simulink model "R2G_ss_NE5kW_R2019a"  (R2019a)
settings: Solver=ode4  StartTime=0  StopTime=1200  FixedStep=simu.dt  MaxStep=0.1  RelTol=1e-3  EnableMultiTasking=on
undefined symbols (not defined in the file or in its folder): ess, gsc, mot, Pgen, Pgrid, Qgrid_lim, simu, Vdc, wsc
libraries: simulink x1
settings Model: Creator=mlawson  LastModifiedBy=eabrowning
settings SolverCC: ZeroCrossControl=DisableAll  AlgebraicLoopSolver=LineSearch  AutoInsertRateTranBlk=on
settings DataIOCC: SaveFormat=Array  SaveOutput=off  SaveTime=off  ReturnWorkspaceOutputs=off
settings OptimizationCC: LifeSpan=inf  SimCompilerOptimization=on
settings DebuggingCC: UnderspecifiedInitializationDetection=Classic  MergeDetectMultiDrivingBlocksExec=none  SolverPrmCheckMsg=warning  AllowSymbolicDim=off  StateNameClashWarn=warning  SFUnexpectedBacktrackingDiag=warning  SFNoUnconditionalDefaultTransitionDiag=warning  ArithmeticOperatorsInVariantConditions=warning
settings HardwareCC: ProdBitPerPointer=32  ProdBitPerSizeT=32  ProdBitPerPtrDiffT=32  ProdLargestAtomicFloat=None  ProdIntDivRoundTo=Undefined  ProdEndianess=Unspecified  ProdWordSize=32  ProdHWDeviceType=32-bit Generic
settings ModelReferenceCC: PropagateSignalLabelsOutOfModel=off
settings SFSimCC: SimUseLocalCustomCode=off
settings RTWCC: RTWUseLocalCustomCode=off
settings CodeAppCC: StateflowObjectComments=on
settings GRTTargetCC: TargetLangStandard=C89/C90 (ANSI)
settings ConfigComp: CovMetricSettings=dw  CovSaveCumulativeToWorkspaceVar=on  CovSaveSingleToWorkspaceVar=on  CovExternalEMLEnable=off  CovSFcnEnable=off
settings SimscapeCC: SimscapeNormalizeSystem=off
settings ConfigurationSet: Description=SimMechanics 2G
settings ExplorerConfigSet: SimMechanicsOpenEditorOnUpdate=off  InternalSimMechanicsExplorerSettings="<ExplorerConfiguration><canonicalview>default</canonicalview><TilePanel><TileInfo><Tiles Columns=\"1\" Count=\"1\" Rows=\"1\"><Column Left=\"2\" Weight=\"1\"/><Column Left=\"1335\"/><Row Top=\"2\" Weight=\"1\"/><Row Top=\"911\"/><Tile Height=\"1\" Width=\"1\" X=\"0\" Y=\"0\"/></Tiles></TileInfo><SceneInfo><SceneViewer><BGColor><R>0.60000002384185791</R><G>0.60000002384185791</G><B>0.60000002384185791</B></BGColor><Camera><Position><X>365.37645888990272</X><Y>-369.82486814446582</Y><Z>359.64809521743916</Z></Position><Center><X>-6.7351450971904585</X><Y>2.2867358426280204</Y><Z>-12.463508769654169</Z></Center><Up><X>-0.40824829046386307</X><Y>0.40824829046386307</Y><Z>0.81649658092772615</Z></Up><Left>-57.820127362122818</Left><Right>57.820127362122818</Right><Bottom>-38.308817187253304</Bottom><Top>38.308817187253304</Top></Camera></SceneViewer></SceneInfo></TilePanel></ExplorerConfiguration>"

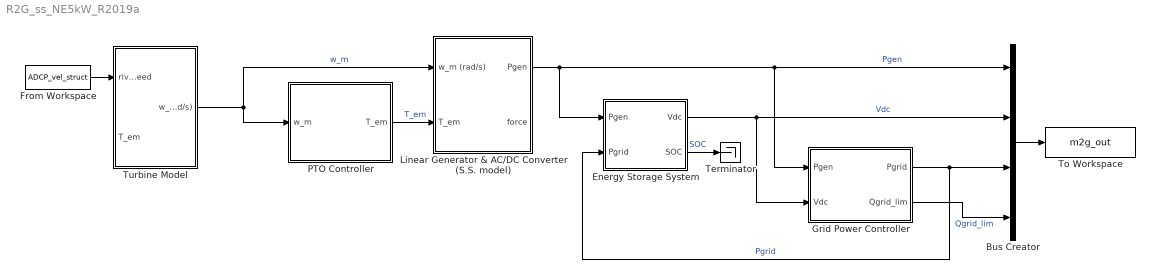
== system R2G_ss_NE5kW_R2019a ==
  Bus Creator : BusCreator  Inputs=Pgen,Vdc,Pgrid,Qgrid_lim
  Energy Storage System : Subsystem  mask{SOC_0=ess.SOC_0, Csoc=ess.Csoc, SOC_LUT=ess.SOC_LUT, Voc_LUT=ess.Voc_LUT, eff=ess.eff}
      mask prompts: SOC_0 "Initial SOC"; Csoc "SOC equivalent capacitance (C):"; SOC_LUT "SOC LUT"; Voc_LUT "Voc LUT"; eff "Efficiency"
      mask DialogControl DescTextVar_copy Prompt: Uses a generalized energy storage model.
      mask DialogControl ParamGroupVar Prompt: Energy Storage Parameters
  From Workspace : FromWorkspace  VariableName=ADCP_vel_struct  OutDataTypeStr=double  OutputAfterFinalValue=Holding final value
  Grid Power Controller : Subsystem  mask{Tavg=gsc.Tavg, Vmag=gsc.Vmag, Ilim=gsc.Ilim, Prated=gsc.Prated, Vdc_nom=ess.Vdc_0, Vdc_del=ess.Vdc_del, kp_v=gsc.kp, ki_v=gsc.ki}
      mask prompts: Tavg "Averaging Time Constant (s):"; Vmag "Grid voltage magnitude (V):"; Ilim "GSC current limit (A):"; Prated "GSC rated power (W):"; Vdc_nom "DC link nominal voltage (V):"; Vdc_del "DC link voltage deviation maximum (V):"; kp_v "Voltage regulator proportional gain:"; ki_v "Voltage regulator integral gain:"
  Linear Generator & AC/DC Converter (S.S. model) : Subsystem  mask{ptoSim=mot}
      mask prompts: ptoSim "Machine Name"
  PTO Controller : Subsystem
  Terminator : Terminator
  To Workspace : ToWorkspace  VariableName=m2g_out  SaveFormat=Timeseries  SampleTime=-1
  Turbine Model : Subsystem
  wires:
  Linear Generator & AC/DC Converter (S.S. model)/1(Pgen) -> Bus Creator/1, Grid Power Controller/1(Pgen), Energy Storage System/1(Pgen)  "Pgen"
  Grid Power Controller/1(Pgrid) -> Bus Creator/3, Energy Storage System/2(Pgrid)  "Pgrid"
  Grid Power Controller/2(Qgrid_lim) -> Bus Creator/4  "Qgrid_lim"
  Energy Storage System/1(Vdc) -> Grid Power Controller/2(Vdc), Bus Creator/2  "Vdc"
  PTO Controller/1(T_em) -> Linear Generator & AC/DC Converter (S.S. model)/2(T_em)  "T_em"
  Bus Creator/1 -> To Workspace/1
  Energy Storage System/2(SOC) -> Terminator/1  "SOC"
  Turbine Model/1(w_m (rad/s)) -> Linear Generator & AC/DC Converter (S.S. model)/1(w_m (rad/s)), PTO Controller/1(w_m)  "w_m"
  From Workspace/1 -> Turbine Model/1(river speed)

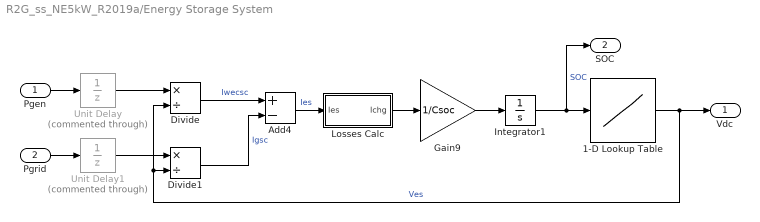
== system R2G_ss_NE5kW_R2019a/Energy Storage System ==
  Pgen : Inport
  Pgrid : Inport  Port=2
  1-D Lookup Table : Lookup_n-D  NumberOfTableDimensions=1  BreakpointsForDimension1=SOC_LUT  Table=Voc_LUT  InternalRulePriority=Speed  RndMeth=Simplest  InputSameDT=on
  Add4 : Sum  Inputs=+-
  Divide : Product  Inputs=*/
  Divide1 : Product  Inputs=*/
  Gain9 : Gain  Gain=1/Csoc
  Integrator1 : Integrator  InitialCondition=SOC_0
  Losses Calc : Subsystem
  Unit Delay : UnitDelay  Commented=through  SampleTime=-1  HasFrameUpgradeWarning=on
  Unit Delay1 : UnitDelay  Commented=through  SampleTime=-1  HasFrameUpgradeWarning=on
  Vdc : Outport  VectorParamsAs1DForOutWhenUnconnected=on
  SOC : Outport  Port=2  VectorParamsAs1DForOutWhenUnconnected=on
  wires:
  Unit Delay1/1 -> Divide1/1
  Unit Delay/1 -> Divide/1
  Pgrid/1 -> Unit Delay1/1
  Divide1/1 -> Add4/2  "Igsc"
  Gain9/1 -> Integrator1/1
  Divide/1 -> Add4/1  "Iwecsc"
  Pgen/1 -> Unit Delay/1
  Integrator1/1 -> SOC/1, 1-D Lookup Table/1  "SOC"
  1-D Lookup Table/1 -> Divide/2, Divide1/2, Vdc/1  "Ves"
  Add4/1 -> Losses Calc/1(Ies)  "Ies"
  Losses Calc/1(Ichg) -> Gain9/1

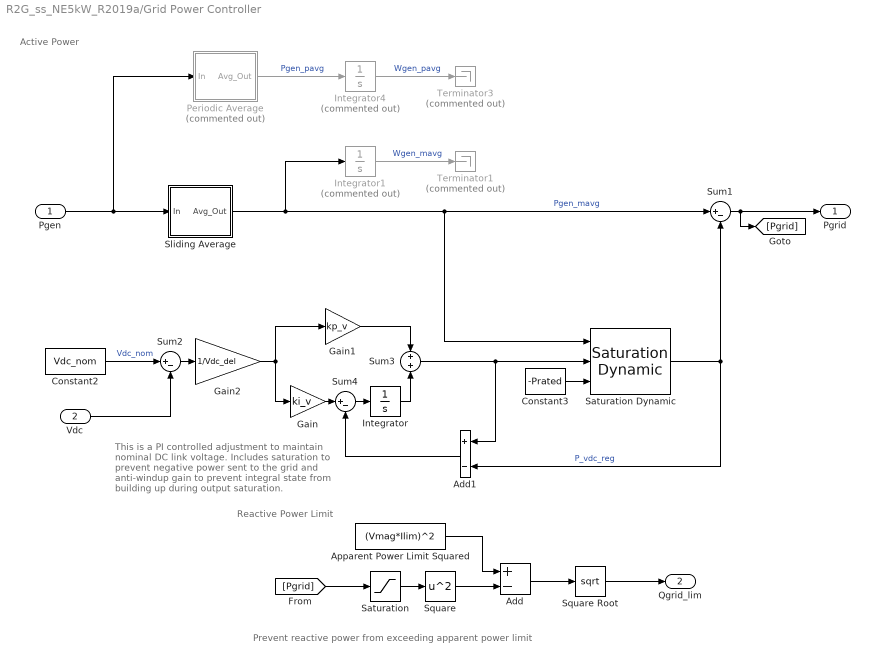
== system R2G_ss_NE5kW_R2019a/Grid Power Controller ==
  note: This is a PI controlled adjustment to maintain nominal DC link voltage. Includes saturation to prevent negative power sent to the grid and anti-windup gain to prevent integral state from building up during output saturation.
  note: Reactive Power Limit
  note: Active Power
  note: Prevent reactive power from exceeding apparent power limit
  Pgen : Inport
  Vdc : Inport  Port=2
  Add : Sum  Inputs=+-
  Add1 : Sum  Inputs=+-
  Apparent Power Limit Squared : Constant  Value=(Vmag*Ilim)^2
  Constant2 : Constant  Value=Vdc_nom
  Constant3 : Constant  Value=-Prated
  Gain : Gain  Gain=ki_v
  Gain1 : Gain  Gain=kp_v
  Gain2 : Gain  Gain=1/Vdc_del
  Integrator : Integrator
  Integrator1 : Integrator  Commented=on
  Integrator4 : Integrator  Commented=on
  Periodic Average : Subsystem  Commented=on  mask{Tsample=Tavg}
      mask prompts: Tsample "Sampling Period (s):"
  Saturation : Saturate  UpperLimit=Vmag*Ilim  LowerLimit=-Vmag*Ilim
  Saturation Dynamic : simulink/Discontinuities/Saturation Dynamic  OutMin=[]  OutMax=[]  OutDataTypeStr=Inherit: Same as second input  OutDataType=fixdt(1, 16)  OutScaling=2^-10  DoSatur=off
  Sliding Average : Subsystem  mask{Tsample=Tavg, dt=simu.dt}
      mask prompts: Tsample "Sampling Period (s):"; dt "Simulation Time Step (s):"
  Square : Math  Operator=square  SaturateOnIntegerOverflow=on
  Square Root : Sqrt  SaturateOnIntegerOverflow=on
  Sum1 : Sum  Inputs=|+-
  Sum2 : Sum  Inputs=|+-
  Sum3 : Sum
  Sum4 : Sum  Inputs=|+-
  Terminator1 : Terminator  Commented=on
  Terminator3 : Terminator  Commented=on
  Pgrid : Outport  VectorParamsAs1DForOutWhenUnconnected=on
  Qgrid_lim : Outport  Port=2  VectorParamsAs1DForOutWhenUnconnected=on
  wires:
  Pgen/1 -> Periodic Average/1(In), Sliding Average/1(In)
  Integrator4/1 -> Terminator3/1  "Wgen_pavg"
  Integrator1/1 -> Terminator1/1  "Wgen_mavg"
  Sliding Average/1(Avg_Out) -> Saturation Dynamic/1, Sum1/1, Integrator1/1  "Pgen_mavg"
  Periodic Average/1(Avg_Out) -> Integrator4/1  "Pgen_pavg"
  Add/1 -> Square Root/1
  Square/1 -> Add/2
  Saturation/1 -> Square/1
  Square Root/1 -> Qgrid_lim/1
  Apparent Power Limit Squared/1 -> Add/1
  Sum1/1 -> [Pgrid], Pgrid/1
  [Pgrid] -> Saturation/1
  Constant2/1 -> Sum2/1  "Vdc_nom"
  Constant3/1 -> Saturation Dynamic/3
  Sum3/1 -> Add1/1, Saturation Dynamic/2
  Gain1/1 -> Sum3/1
  Integrator/1 -> Sum3/2
  Saturation Dynamic/1 -> Add1/2, Sum1/2  "P_vdc_reg"
  Vdc/1 -> Sum2/2
  Sum2/1 -> Gain2/1
  Gain2/1 -> Gain1/1, Gain/1
  Gain/1 -> Sum4/1
  Sum4/1 -> Integrator/1
  Add1/1 -> Sum4/2

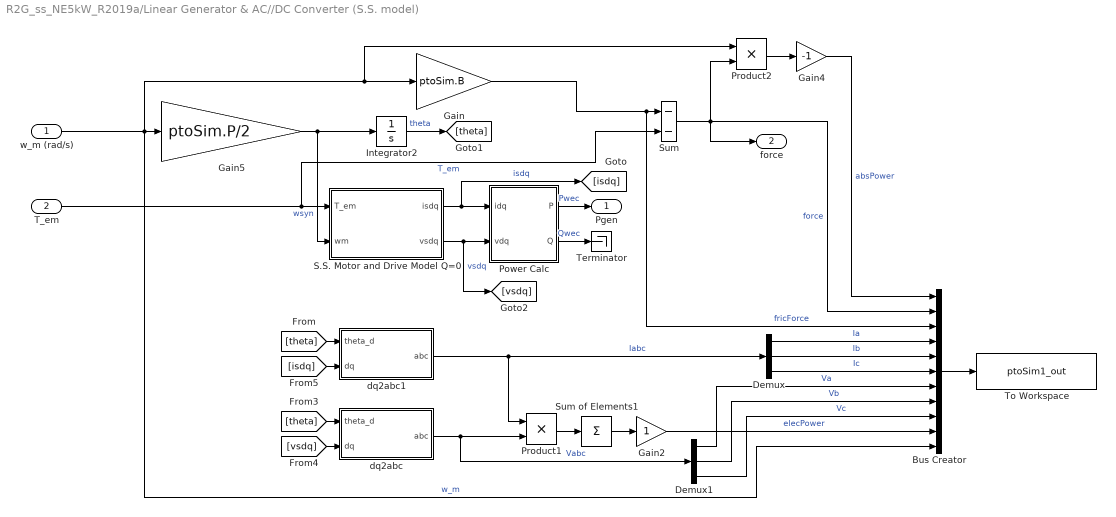
== system R2G_ss_NE5kW_R2019a/Linear Generator & AC//DC Converter (S.S. model) ==
  w_m (rad/s) : Inport
  T_em : Inport  Port=2
  Bus Creator : BusCreator  Inputs=11
  Demux : Demux  Outputs=3
  Demux1 : Demux  Outputs=3
  Gain : Gain  Gain=ptoSim.B
  Gain2 : Gain
  Gain4 : Gain  Gain=-1
  Gain5 : Gain  Gain=ptoSim.P/2
  Integrator2 : Integrator  InitialCondition=ptoSim.theta_d_0
  Power Calc : Subsystem
  Product1 : Product
  Product2 : Product
  S.S. Motor and Drive Model Q=0 : Subsystem
  Sum : Sum  Inputs=--
  Sum of Elements1 : Sum  Inputs=+
  Terminator : Terminator
  To Workspace : ToWorkspace  VariableName=ptoSim1_out  SaveFormat=Structure With Time  SampleTime=simu.dt
  dq2abc : Subsystem
  dq2abc1 : Subsystem
  Pgen : Outport  VectorParamsAs1DForOutWhenUnconnected=on
  force : Outport  Port=2  VectorParamsAs1DForOutWhenUnconnected=on
  wires:
  Gain/1 -> Sum/1, Bus Creator/3  "fricForce"
  S.S. Motor and Drive Model Q=0/2(vsdq) -> [vsdq], Power Calc/2(vdq)  "vsdq"
  Sum/1 -> Product2/2, force/1, Bus Creator/2  "force"
  Sum of Elements1/1 -> Gain2/1
  Integrator2/1 -> [theta]  "theta"
  w_m (rad/s)/1 -> Gain/1, Product2/1, Bus Creator/11, Gain5/1  "w_m"
  Gain2/1 -> Bus Creator/10  "elecPower"
  Product1/1 -> Sum of Elements1/1
  dq2abc/1(abc) -> Demux1/1, Product1/2  "Vabc"
  Demux1/3 -> Bus Creator/9  "Vc"
  Demux1/2 -> Bus Creator/8  "Vb"
  Demux/3 -> Bus Creator/6  "Ic"
  Gain5/1 -> Integrator2/1, S.S. Motor and Drive Model Q=0/2(wm)  "wsyn"
  Demux1/1 -> Bus Creator/7  "Va"
  Demux/1 -> Bus Creator/4  "Ia"
  S.S. Motor and Drive Model Q=0/1(isdq) -> Power Calc/1(idq), [isdq]  "isdq"
  Bus Creator/1 -> To Workspace/1
  Demux/2 -> Bus Creator/5  "Ib"
  dq2abc1/1(abc) -> Product1/1, Demux/1  "Iabc"
  Gain4/1 -> Bus Creator/1  "absPower"
  Product2/1 -> Gain4/1
  Power Calc/2(Q) -> Terminator/1  "Qwec"
  Power Calc/1(P) -> Pgen/1  "Pwec"
  [theta] -> dq2abc1/1(theta_d)
  [theta] -> dq2abc/1(theta_d)
  [vsdq] -> dq2abc/2(dq)
  [isdq] -> dq2abc1/2(dq)
  T_em/1 -> S.S. Motor and Drive Model Q=0/1(T_em), Sum/2  "T_em"

== system R2G_ss_NE5kW_R2019a/PTO Controller ==
  w_m : Inport
  Current-based force limit : Saturate  UpperLimit=wsc.Fpto_lim  LowerLimit=-wsc.Fpto_lim
  Gain1 : Gain  Gain=wsc.Bdamp
  T_em : Outport  VectorParamsAs1DForOutWhenUnconnected=on
  wires:
  Gain1/1 -> Current-based force limit/1  "T_em"
  w_m/1 -> Gain1/1
  Current-based force limit/1 -> T_em/1

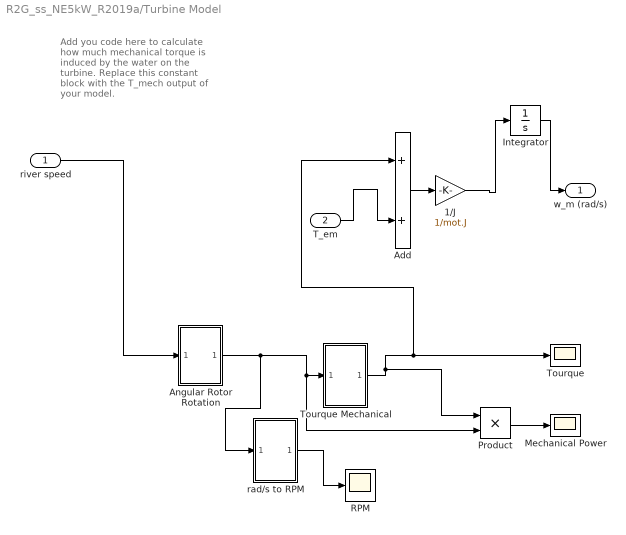
== system R2G_ss_NE5kW_R2019a/Turbine Model ==
  note: Add you code here to calculate how much mechanical torque is induced by the water on the turbine. Replace this constant block with the T_mech output of your model.
  river speed : Inport
  T_em : Inport  Port=2
  " Tourque Mechanical" : Subsystem
  1/J : Gain  Gain=1/mot.J
  Add : Sum
  Angular Rotor Rotation : Subsystem
  Integrator : Integrator
  Mechanical Power : Scope
  Product : Product
  RPM : Scope
  Tourque : Scope
  rad/s to RPM : Subsystem
  w_m (rad/s) : Outport  VectorParamsAs1DForOutWhenUnconnected=on
  wires:
  1/J/1 -> Integrator/1
  Add/1 -> 1/J/1
  rad/s to RPM/1(Out1) -> RPM/1
  Angular Rotor Rotation/1(Out1) -> rad/s to RPM/1(In1), Product/2, " Tourque Mechanical"/1(In1)
  river speed/1 -> Angular Rotor Rotation/1(In1)
  Product/1 -> Mechanical Power/1
  " Tourque Mechanical"/1(Out1) -> Add/1, Tourque/1, Product/1
  T_em/1 -> Add/2
  Integrator/1 -> w_m (rad/s)/1

== system R2G_ss_NE5kW_R2019a/Energy Storage System/Losses Calc ==
  Ies : Inport
  Gain1 : Gain  Gain=1/eff
  Gain2 : Gain  Gain=eff
  Switch : Switch  Criteria=u2 > Threshold
  Ichg : Outport  VectorParamsAs1DForOutWhenUnconnected=on
  wires:
  Ies/1 -> Gain1/1, Gain2/1, Switch/2
  Switch/1 -> Ichg/1
  Gain2/1 -> Switch/1
  Gain1/1 -> Switch/3

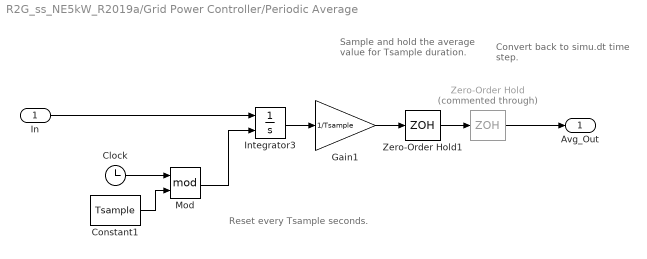
== system R2G_ss_NE5kW_R2019a/Grid Power Controller/Periodic Average ==
  note: Reset every Tsample seconds.
  note: Convert back to simu.dt time step.
  note: Sample and hold the average value for Tsample duration.
  In : Inport
  Clock : Clock
  Constant1 : Constant  Value=Tsample
  Gain1 : Gain  Gain=1/Tsample
  Integrator3 : Integrator  ExternalReset=rising
  Mod : Math  Operator=mod  OutputSignalType=real  SaturateOnIntegerOverflow=on
  Zero-Order Hold : ZeroOrderHold  Commented=through  SampleTime=simu.dt
  Zero-Order Hold1 : ZeroOrderHold  SampleTime=Tsample
  Avg_Out : Outport  VectorParamsAs1DForOutWhenUnconnected=on
  wires:
  Zero-Order Hold/1 -> Avg_Out/1
  Mod/1 -> Integrator3/2
  Zero-Order Hold1/1 -> Zero-Order Hold/1
  Clock/1 -> Mod/1
  Gain1/1 -> Zero-Order Hold1/1
  Integrator3/1 -> Gain1/1
  In/1 -> Integrator3/1
  Constant1/1 -> Mod/2

== system R2G_ss_NE5kW_R2019a/Grid Power Controller/Sliding Average ==
  In : Inport
  Discrete FIR Filter : DiscreteFir  Coefficients=ones(1,round(Tsample/dt))/round(Tsample/dt)  SampleTime=dt
  Avg_Out : Outport  VectorParamsAs1DForOutWhenUnconnected=on
  wires:
  In/1 -> Discrete FIR Filter/1
  Discrete FIR Filter/1 -> Avg_Out/1

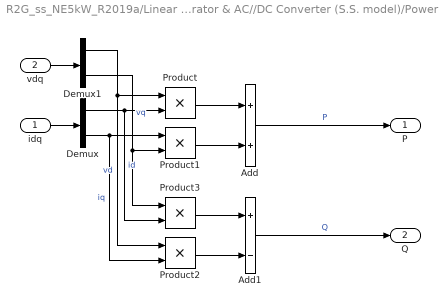
== system R2G_ss_NE5kW_R2019a/Linear Generator & AC//DC Converter (S.S. model)/Power Calc ==
  idq : Inport
  vdq : Inport  Port=2
  Add : Sum
  Add1 : Sum  Inputs=+-
  Demux : Demux  Outputs=2
  Demux1 : Demux  Outputs=2
  Product{,1..3} (4 alike) : Product
  P : Outport  VectorParamsAs1DForOutWhenUnconnected=on
  Q : Outport  Port=2  VectorParamsAs1DForOutWhenUnconnected=on
  wires:
  Demux/1 -> Product3/2, Product/2  "id"
  Product1/1 -> Add/2
  Add1/1 -> Q/1  "Q"
  Demux1/2 -> Product1/2, Product3/1  "vq"
  Demux1/1 -> Product/1, Product2/1  "vd"
  Demux/2 -> Product2/2, Product1/1  "iq"
  Product3/1 -> Add1/1
  Product2/1 -> Add1/2
  Product/1 -> Add/1
  Add/1 -> P/1  "P"
  idq/1 -> Demux/1
  vdq/1 -> Demux1/1

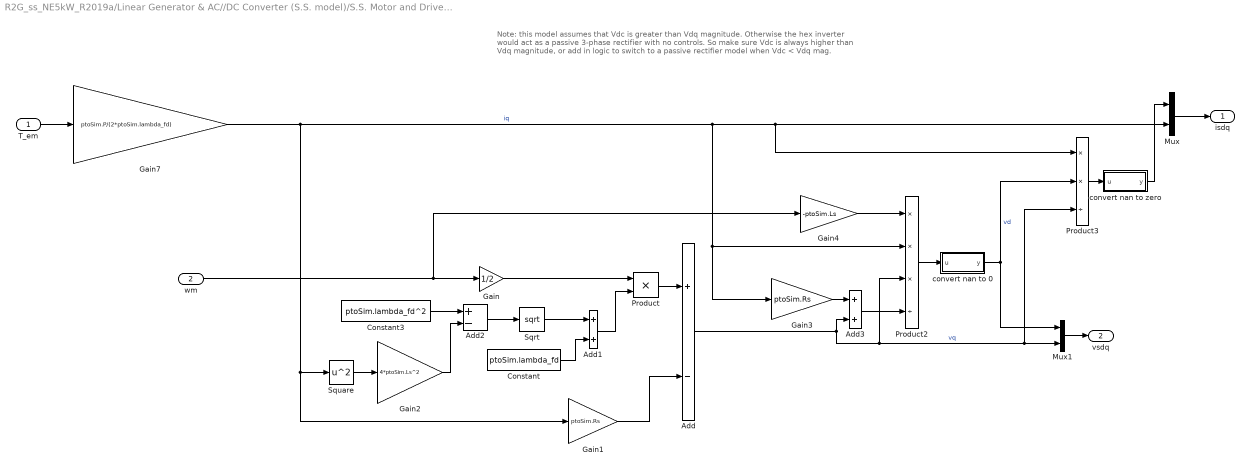
== system R2G_ss_NE5kW_R2019a/Linear Generator & AC//DC Converter (S.S. model)/S.S. Motor and Drive Model Q=0 ==
  note: Note: this model assumes that Vdc is greater than Vdq magnitude. Otherwise the hex inverter would act as a passive 3-phase rectifier with no controls. So make sure Vdc is always higher than Vdq magnitude, or add in logic to switch to a passive rectifier model when Vdc < Vdq mag.
  T_em : Inport
  wm : Inport  Port=2
  Add : Sum  Inputs=+-
  Add1 : Sum
  Add2 : Sum  Inputs=+-
  Add3 : Sum
  Constant : Constant  Value=ptoSim.lambda_fd
  Constant3 : Constant  Value=ptoSim.lambda_fd^2
  Gain : Gain  Gain=1/2
  Gain1 : Gain  Gain=ptoSim.Rs
  Gain2 : Gain  Gain=4*ptoSim.Ls^2
  Gain3 : Gain  Gain=ptoSim.Rs
  Gain4 : Gain  Gain=-ptoSim.Ls
  Gain7 : Gain  Gain=ptoSim.P/(2*ptoSim.lambda_fd)
  Mux : Mux  Inputs=2
  Mux1 : Mux  Inputs=2
  Product : Product
  Product2 : Product  Inputs=***/
  Product3 : Product  Inputs=**/
  Sqrt : Sqrt  SaturateOnIntegerOverflow=on
  Square : Math  Operator=square  SaturateOnIntegerOverflow=on
  convert nan to 0 : MATLAB Function  TreatAsAtomicUnit=on
  convert nan to zero : MATLAB Function  TreatAsAtomicUnit=on
  isdq : Outport  VectorParamsAs1DForOutWhenUnconnected=on
  vsdq : Outport  Port=2  VectorParamsAs1DForOutWhenUnconnected=on
  wires:
  T_em/1 -> Gain7/1
  Mux/1 -> isdq/1
  Mux1/1 -> vsdq/1
  Gain7/1 -> Product2/2, Gain3/1, Product3/1, Mux/2, Gain1/1, Square/1  "iq"
  Constant/1 -> Add1/2
  convert nan to 0/1(y) -> Product3/2, Mux1/1  "vd"
  Add/1 -> Product2/3, Product3/3, Mux1/2, Add3/2  "vq"
  convert nan to zero/1(y) -> Mux/1
  Gain1/1 -> Add/2
  Product/1 -> Add/1
  Gain/1 -> Product/1
  Add1/1 -> Product/2
  Sqrt/1 -> Add1/1
  Add2/1 -> Sqrt/1
  Constant3/1 -> Add2/1
  Gain2/1 -> Add2/2
  Product2/1 -> convert nan to 0/1(u)
  Add3/1 -> Product2/4
  Gain3/1 -> Add3/1
  Gain4/1 -> Product2/1
  Product3/1 -> convert nan to zero/1(u)
  Square/1 -> Gain2/1
  wm/1 -> Gain4/1, Gain/1

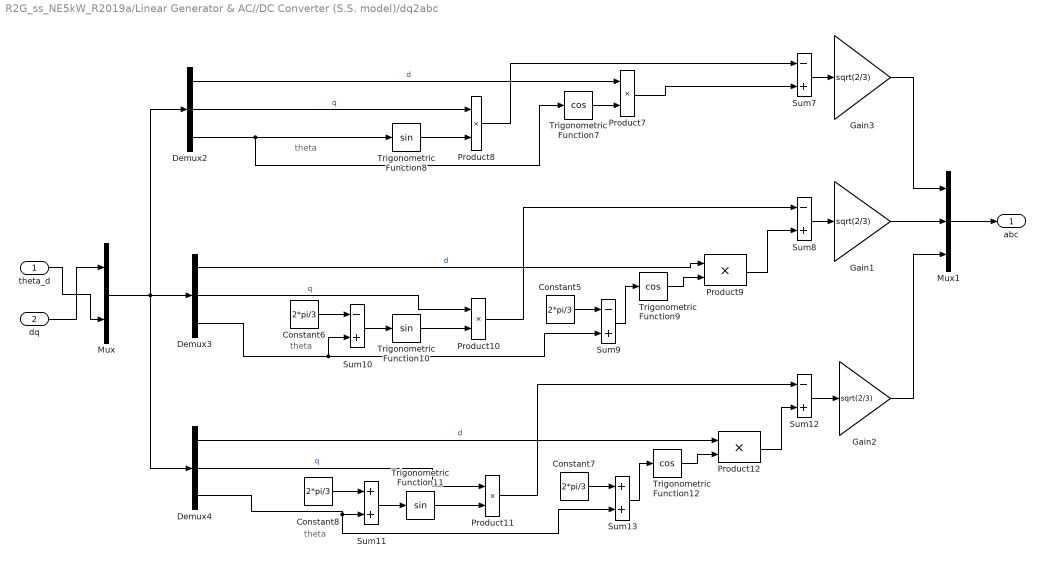
== system R2G_ss_NE5kW_R2019a/Linear Generator & AC//DC Converter (S.S. model)/dq2abc ==
  note: theta
  note: theta
  note: theta
  theta_d : Inport
  dq : Inport  Port=2
  Constant{5..8} (4 alike) : Constant  Value=2*pi/3
  Demux2 : Demux  Outputs=3
  Demux3 : Demux  Outputs=3
  Demux4 : Demux  Outputs=3
  Gain1 : Gain  Gain=sqrt(2/3)  SaturateOnIntegerOverflow=on  OutDataTypeStr=Inherit: Same as input  ParamDataTypeStr=Inherit: Same as input
  Gain2 : Gain  Gain=sqrt(2/3)  SaturateOnIntegerOverflow=on  OutDataTypeStr=Inherit: Same as input  ParamDataTypeStr=Inherit: Same as input
  Gain3 : Gain  Gain=sqrt(2/3)  SaturateOnIntegerOverflow=on  OutDataTypeStr=Inherit: Same as input  ParamDataTypeStr=Inherit: Same as input
  Mux : Mux  Inputs=2
  Mux1 : Mux  Inputs=3
  Product{7..12} (6 alike) : Product  SaturateOnIntegerOverflow=on  InputSameDT=on  OutDataTypeStr=Inherit: Same as first input
  Sum{7..10,12} (5 alike) : Sum  Inputs=-+  SaturateOnIntegerOverflow=on  InputSameDT=on  OutDataTypeStr=Inherit: Same as first input
  Sum11 : Sum  SaturateOnIntegerOverflow=on  InputSameDT=on  OutDataTypeStr=Inherit: Same as first input
  Sum13 : Sum  SaturateOnIntegerOverflow=on  InputSameDT=on  OutDataTypeStr=Inherit: Same as first input
  Trigonometric Function10 : Trigonometry
  Trigonometric Function11 : Trigonometry
  Trigonometric Function12 : Trigonometry  Operator=cos
  Trigonometric Function7 : Trigonometry  Operator=cos
  Trigonometric Function8 : Trigonometry
  Trigonometric Function9 : Trigonometry  Operator=cos
  abc : Outport  VectorParamsAs1DForOutWhenUnconnected=on
  wires:
  Constant8/1 -> Sum11/1
  Product7/1 -> Sum7/2
  Gain1/1 -> Mux1/2
  Product9/1 -> Sum8/2
  Sum7/1 -> Gain3/1
  Demux4/2 -> Product11/1  "q"
  Product10/1 -> Sum8/1
  Product11/1 -> Sum12/1
  Sum13/1 -> Trigonometric Function12/1
  Demux2/3 -> Trigonometric Function7/1, Trigonometric Function8/1
  Product12/1 -> Sum12/2
  Constant6/1 -> Sum10/1
  Product8/1 -> Sum7/1
  Mux1/1 -> abc/1
  Demux3/3 -> Sum9/2, Sum10/2
  Demux3/2 -> Product10/1  "q"
  Demux2/2 -> Product8/1  "q"
  dq/1 -> Mux/1
  Trigonometric Function7/1 -> Product7/2
  Constant5/1 -> Sum9/1
  Trigonometric Function12/1 -> Product12/2
  Trigonometric Function10/1 -> Product10/2
  Demux4/1 -> Product12/1  "d"
  Gain2/1 -> Mux1/3
  Demux4/3 -> Sum11/2, Sum13/2
  Demux2/1 -> Product7/1  "d"
  Sum10/1 -> Trigonometric Function10/1
  Gain3/1 -> Mux1/1
  Mux/1 -> Demux3/1, Demux2/1, Demux4/1
  Sum12/1 -> Gain2/1
  theta_d/1 -> Mux/2
  Sum11/1 -> Trigonometric Function11/1
  Trigonometric Function9/1 -> Product9/2
  Sum8/1 -> Gain1/1
  Sum9/1 -> Trigonometric Function9/1
  Demux3/1 -> Product9/1  "d"
  Trigonometric Function8/1 -> Product8/2
  Trigonometric Function11/1 -> Product11/2
  Constant7/1 -> Sum13/1

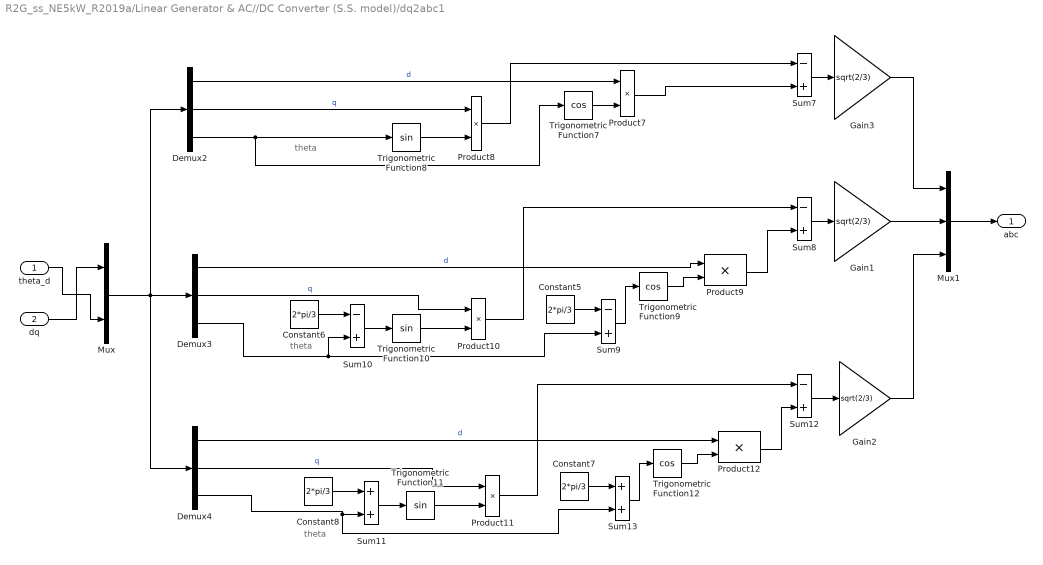
== system R2G_ss_NE5kW_R2019a/Linear Generator & AC//DC Converter (S.S. model)/dq2abc1 ==
  note: theta
  note: theta
  note: theta
  theta_d : Inport
  dq : Inport  Port=2
  Constant{5..8} (4 alike) : Constant  Value=2*pi/3
  Demux2 : Demux  Outputs=3
  Demux3 : Demux  Outputs=3
  Demux4 : Demux  Outputs=3
  Gain1 : Gain  Gain=sqrt(2/3)  SaturateOnIntegerOverflow=on  OutDataTypeStr=Inherit: Same as input  ParamDataTypeStr=Inherit: Same as input
  Gain2 : Gain  Gain=sqrt(2/3)  SaturateOnIntegerOverflow=on  OutDataTypeStr=Inherit: Same as input  ParamDataTypeStr=Inherit: Same as input
  Gain3 : Gain  Gain=sqrt(2/3)  SaturateOnIntegerOverflow=on  OutDataTypeStr=Inherit: Same as input  ParamDataTypeStr=Inherit: Same as input
  Mux : Mux  Inputs=2
  Mux1 : Mux  Inputs=3
  Product{7..12} (6 alike) : Product  SaturateOnIntegerOverflow=on  InputSameDT=on  OutDataTypeStr=Inherit: Same as first input
  Sum{7..10,12} (5 alike) : Sum  Inputs=-+  SaturateOnIntegerOverflow=on  InputSameDT=on  OutDataTypeStr=Inherit: Same as first input
  Sum11 : Sum  SaturateOnIntegerOverflow=on  InputSameDT=on  OutDataTypeStr=Inherit: Same as first input
  Sum13 : Sum  SaturateOnIntegerOverflow=on  InputSameDT=on  OutDataTypeStr=Inherit: Same as first input
  Trigonometric Function10 : Trigonometry
  Trigonometric Function11 : Trigonometry
  Trigonometric Function12 : Trigonometry  Operator=cos
  Trigonometric Function7 : Trigonometry  Operator=cos
  Trigonometric Function8 : Trigonometry
  Trigonometric Function9 : Trigonometry  Operator=cos
  abc : Outport  VectorParamsAs1DForOutWhenUnconnected=on
  wires:
  Constant8/1 -> Sum11/1
  Product7/1 -> Sum7/2
  Gain1/1 -> Mux1/2
  Product9/1 -> Sum8/2
  Sum7/1 -> Gain3/1
  Demux4/2 -> Product11/1  "q"
  Product10/1 -> Sum8/1
  Product11/1 -> Sum12/1
  Sum13/1 -> Trigonometric Function12/1
  Demux2/3 -> Trigonometric Function7/1, Trigonometric Function8/1
  Product12/1 -> Sum12/2
  Constant6/1 -> Sum10/1
  Product8/1 -> Sum7/1
  Mux1/1 -> abc/1
  Demux3/3 -> Sum9/2, Sum10/2
  Demux3/2 -> Product10/1  "q"
  Demux2/2 -> Product8/1  "q"
  dq/1 -> Mux/1
  Trigonometric Function7/1 -> Product7/2
  Constant5/1 -> Sum9/1
  Trigonometric Function12/1 -> Product12/2
  Trigonometric Function10/1 -> Product10/2
  Demux4/1 -> Product12/1  "d"
  Gain2/1 -> Mux1/3
  Demux4/3 -> Sum11/2, Sum13/2
  Demux2/1 -> Product7/1  "d"
  Sum10/1 -> Trigonometric Function10/1
  Gain3/1 -> Mux1/1
  Mux/1 -> Demux3/1, Demux2/1, Demux4/1
  Sum12/1 -> Gain2/1
  theta_d/1 -> Mux/2
  Sum11/1 -> Trigonometric Function11/1
  Trigonometric Function9/1 -> Product9/2
  Sum8/1 -> Gain1/1
  Sum9/1 -> Trigonometric Function9/1
  Demux3/1 -> Product9/1  "d"
  Trigonometric Function8/1 -> Product8/2
  Trigonometric Function11/1 -> Product11/2
  Constant7/1 -> Sum13/1

== system R2G_ss_NE5kW_R2019a/Turbine Model/ Tourque Mechanical ==
  In1 : Inport
  Product : Product
  Square : Math  Operator=square  SaturateOnIntegerOverflow=on
  specific constant kgm^2 : Constant  Value=5.97
  Out1 : Outport
  wires:
  In1/1 -> Square/1
  Square/1 -> Product/1
  specific constant kgm^2/1 -> Product/2
  Product/1 -> Out1/1

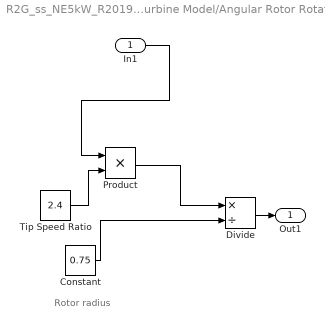
== system R2G_ss_NE5kW_R2019a/Turbine Model/Angular Rotor Rotation ==
  note: Rotor radius
  In1 : Inport
  Constant : Constant  Value=0.75
  Divide : Product  Inputs=*/
  Product : Product
  "Tip Speed Ratio " : Constant  Value=2.4
  Out1 : Outport
  wires:
  Constant/1 -> Divide/2
  "Tip Speed Ratio "/1 -> Product/2
  In1/1 -> Product/1
  Divide/1 -> Out1/1
  Product/1 -> Divide/1

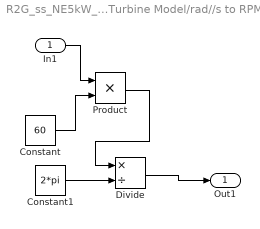
== system R2G_ss_NE5kW_R2019a/Turbine Model/rad//s to RPM ==
  In1 : Inport
  Constant : Constant  Value=60
  Constant1 : Constant  Value=2*pi
  Divide : Product  Inputs=*/
  Product : Product
  Out1 : Outport
  wires:
  Constant/1 -> Product/2
  Product/1 -> Divide/1
  Divide/1 -> Out1/1
  Constant1/1 -> Divide/2
  In1/1 -> Product/1

== matlab function R2G_ss_NE5kW_R2019a/Linear Generator & AC//DC Converter (S.S. model)/S.S. Motor and Drive Model Q=0/convert nan to 0 ==
  data: u input; y output
function y = fcn(u)
if isnan(u)
    y=0;
else
    y = u;
end
end

== matlab function R2G_ss_NE5kW_R2019a/Linear Generator & AC//DC Converter (S.S. model)/S.S. Motor and Drive Model Q=0/convert nan to zero ==
  data: u input; y output
function y = fcn(u)
if isnan(u)
    y=0;
else
    y = u;
end
end
